simulink model "prve_riadenie"  (Simulink 7.4)
settings: Solver=ode4  StartTime=0.0  StopTime=t_sim  FixedStep=Ts  RelTol=1e-3
values from neighbouring files (symbols this model uses):
  baud = 115200    [test.m]
  com = '/dev/ttyACM0,output2.txt'    [test.m]
  D = 0    [test.m]
  fTf = 0.5    [test.m]
  fTl = 0.5    [test.m]
  fTt = 0.5    [test.m]
  I = 0    [test.m]
  P = 0    [test.m]
  Ts = 0.02    [test.m]
undefined symbols (not defined in the file or in its folder): cfan, clamp, cled, ctrltyp, insw, outsw, vstup
libraries: simulink x1, tos_lib x1
settings Model: Creator=tom  LastModifiedBy=moje
settings DataIOCC: LimitDataPoints=off  SaveOutput=off  SignalLogging=off  SaveTime=off
settings DebuggingCC: AlgebraicLoopMsg=none  ArtificialAlgebraicLoopMsg=none

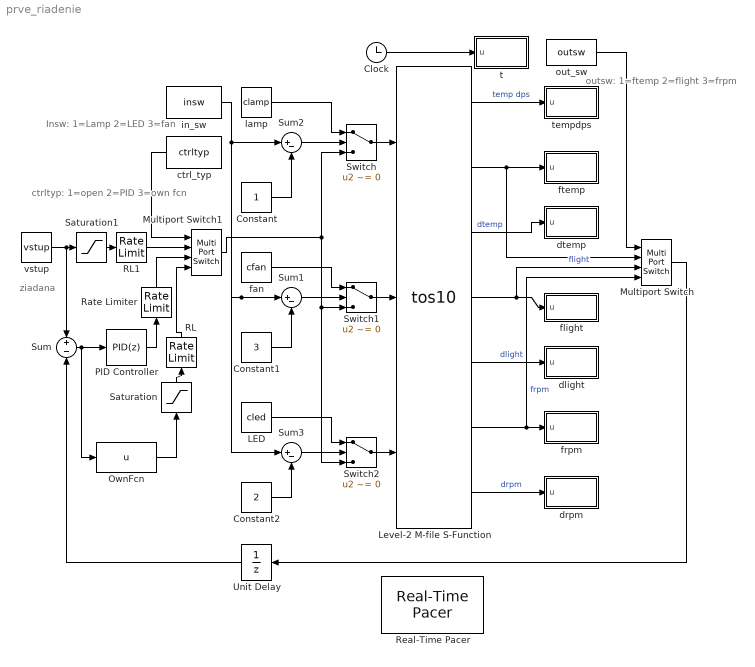
== system prve_riadenie ==
  note: ziadana
  note: Insw:
      | 1=Lamp
      | 2=LED
      | 3=fan
  note: outsw:
      | 1=ftemp
      | 2=flight
      | 3=frpm
  note: ctrltyp:
      | 1=open
      | 2=PID
      | 3=own fcn
  Clock : Clock
      settings: Decimation=10
  Constant : Constant  OutDataType=fixdt(1, 16)  OutScaling=2^0  SampleTime=Ts
  Constant1 : Constant  Value=3  OutDataType=fixdt(1, 16)  OutScaling=2^0  SampleTime=Ts
  Constant2 : Constant  Value=2  OutDataType=fixdt(1, 16)  OutScaling=2^0  SampleTime=Ts
  LED : Constant  Value=cled  SampleTime=Ts
  Level-2 M-file S-Function : M-S-Function  FunctionName=tos10  Parameters=Ts,com,baud,fTt,fTl,fTf
  Multiport Switch : MultiPortSwitch  OutDataTypeMode=double  OutDataType=fixdt(1, 16)  OutScaling=2^0  OutDataTypeStr=double  SampleTime=Ts
  Multiport Switch1 : MultiPortSwitch  OutDataTypeMode=double  OutDataType=fixdt(1, 16)  OutScaling=2^0  OutDataTypeStr=double  SampleTime=Ts
  OwnFcn : Fcn  Expr=u  SampleTime=Ts
  PID Controller : simulink/Continuous/PID Controller  DialogController=pidpack.PIDConfig.pidDDGCreate  DialogControllerArgs=DataTag0  SystemSampleTime=-1  Controller=PID  TimeDomain=Discrete-time  SampleTime=Ts  IntegratorMethod=Forward Euler  FilterMethod=Forward Euler  Form=Parallel  P=P  I=I  D=D  N=10  InitialConditionSource=internal  InitialConditionForIntegrator=0  InitialConditionForFilter=0  ExternalReset=none  LimitOutput=on  UpperSaturationLimit=100  LowerSaturationLimit=0  LinearizeAsGain=off  AntiWindupMode=clamping  Kb=10  TrackingMode=off  Kt=1  PParamMin=[]  PParamMax=[]  IParamMin=[]  IParamMax=[]  DParamMin=[]  DParamMax=[]  NParamMin=[]  NParamMax=[]  KbParamMin=[]  KbParamMax=[]  KtParamMin=[]  KtParamMax=[]  POutMin=[]  POutMax=[]  IOutMin=[]  IOutMax=[]  DOutMin=[]  DOutMax=[]  NOutMin=[]  NOutMax=[]  KbOutMin=[]  KbOutMax=[]  KtOutMin=[]  KtOutMax=[]  IntegratorOutMin=[]  IntegratorOutMax=[]  FilterOutMin=[]  FilterOutMax=[]  SumOutMin=[]  SumOutMax=[]  SumI1OutMin=[]  SumI1OutMax=[]  SumI1OutDataTypeStr=single  SumI2OutMin=[]  SumI2OutMax=[]  SumI3OutMin=[]  SumI3OutMax=[]  SumDOutMin=[]  SumDOutMax=[]  SaturationOutMin=[]  SaturationOutMax=[]  IntegratorContinuousStateAttributes=''  IntegratorStateMustResolveToSignalObject=off  IntegratorRTWStateStorageClass=Auto  FilterContinuousStateAttributes=''  FilterStateMustResolveToSignalObject=off  FilterRTWStateStorageClass=Auto
  RL : RateLimiter  RisingSlewLimit=10  FallingSlewLimit=-10  SampleTimeMode=inherited
  RL1 : RateLimiter  RisingSlewLimit=10  FallingSlewLimit=-10  SampleTimeMode=inherited
  Rate Limiter : RateLimiter  RisingSlewLimit=10  FallingSlewLimit=-10  SampleTimeMode=inherited
  Real-Time Pacer : tos_lib/Real-Time Pacer  simTimePerRealTime=1
  Saturation : Saturate  UpperLimit=100  LowerLimit=0  SampleTime=Ts  OutDataType=fixdt(1, 16)  OutScaling=2^0
  Saturation1 : Saturate  UpperLimit=100  LowerLimit=0  SampleTime=Ts  OutDataType=fixdt(1, 16)  OutScaling=2^0
  Sum : Sum  Inputs=+|-  OutDataType=fixdt(1, 16)  OutScaling=2^0  SampleTime=Ts
  Sum1 : Sum  Inputs=|+-  OutDataType=fixdt(1, 16)  OutScaling=2^0  SampleTime=Ts
  Sum2 : Sum  Inputs=|+-  OutDataType=fixdt(1, 16)  OutScaling=2^0  SampleTime=Ts
  Sum3 : Sum  Inputs=|+-  OutDataType=fixdt(1, 16)  OutScaling=2^0  SampleTime=Ts
  Switch : Switch  Criteria=u2 ~= 0  OutDataTypeMode=double  OutDataType=fixdt(1, 16)  OutScaling=2^0  OutDataTypeStr=double
  Switch1 : Switch  Criteria=u2 ~= 0  OutDataTypeMode=double  OutDataType=fixdt(1, 16)  OutScaling=2^0  OutDataTypeStr=double
  Switch2 : Switch  Criteria=u2 ~= 0  OutDataTypeMode=double  OutDataType=fixdt(1, 16)  OutScaling=2^0  OutDataTypeStr=double  SampleTime=Ts
  Unit Delay : UnitDelay  SampleTime=Ts
  ctrl_typ : Constant  Value=ctrltyp  SampleTime=Ts
  dlight : Stateflow chart  TreatAsAtomicUnit=on  SystemSampleTime=Ts
  drpm : Stateflow chart  TreatAsAtomicUnit=on  SystemSampleTime=Ts
  dtemp : Stateflow chart  TreatAsAtomicUnit=on  SystemSampleTime=Ts
  fan : Constant  Value=cfan  SampleTime=Ts
  flight : Stateflow chart  TreatAsAtomicUnit=on  SystemSampleTime=Ts
  frpm : Stateflow chart  TreatAsAtomicUnit=on  SystemSampleTime=Ts
  ftemp : Stateflow chart  TreatAsAtomicUnit=on  SystemSampleTime=Ts
  in_sw : Constant  Value=insw  SampleTime=Ts
  lamp : Constant  Value=clamp  SampleTime=Ts
  out_sw : Constant  Value=outsw  SampleTime=Ts
  t : Stateflow chart  TreatAsAtomicUnit=on  SystemSampleTime=Ts
  tempdps : Stateflow chart  TreatAsAtomicUnit=on  SystemSampleTime=Ts
  vstup : Constant  Value=vstup  SampleTime=Ts
  wires:
  lamp/1 -> Switch/1
  fan/1 -> Switch1/1
  LED/1 -> Switch2/1
  Switch/1 -> Level-2 M-file S-Function/1
  Switch1/1 -> Level-2 M-file S-Function/2
  Switch2/1 -> Level-2 M-file S-Function/3
  Sum3/1 -> Switch2/2
  Sum1/1 -> Switch1/2
  Sum2/1 -> Switch/2
  in_sw/1 -> Sum2/1, Sum1/1, Sum3/1
  Constant/1 -> Sum2/2
  Constant1/1 -> Sum1/2
  Constant2/1 -> Sum3/2
  Multiport Switch1/1 -> Switch/3, Switch1/3, Switch2/3
  vstup/1 -> Sum/1, Saturation1/1
  PID Controller/1 -> Rate Limiter/1
  Sum/1 -> PID Controller/1, OwnFcn/1
  Clock/1 -> t/1(u)
  Level-2 M-file S-Function/4 -> Multiport Switch/3, flight/1(u)  "flight"
  Level-2 M-file S-Function/5 -> dlight/1(u)  "dlight"
  Level-2 M-file S-Function/7 -> drpm/1(u)  "drpm"
  Level-2 M-file S-Function/6 -> Multiport Switch/4, frpm/1(u)  "frpm"
  Level-2 M-file S-Function/2 -> ftemp/1(u), Multiport Switch/2
  Level-2 M-file S-Function/3 -> dtemp/1(u)  "dtemp"
  Level-2 M-file S-Function/1 -> tempdps/1(u)  "temp dps"
  out_sw/1 -> Multiport Switch/1
  Multiport Switch/1 -> Unit Delay/1
  Unit Delay/1 -> Sum/2
  Rate Limiter/1 -> Multiport Switch1/3
  RL/1 -> Multiport Switch1/4
  Saturation/1 -> RL/1
  OwnFcn/1 -> Saturation/1
  ctrl_typ/1 -> Multiport Switch1/1
  Saturation1/1 -> RL1/1
  RL1/1 -> Multiport Switch1/2

== matlab function ftemp ==
  data: u input double
function fcn(u)
%#eml
eml.extrinsic('num2str');
eml.extrinsic('strcat');
eml.extrinsic('evalin');
evalin('base',strcat('ftemp(end+1)=', num2str(u),';'));
end

== matlab function tempdps ==
  data: u input double
function fcn(u)
%#eml
eml.extrinsic('num2str');
eml.extrinsic('strcat');
eml.extrinsic('evalin');
evalin('base',strcat('tempdps(end+1)=', num2str(u),';'));
end

== matlab function dtemp ==
  data: u input double
function fcn(u)
%#eml
eml.extrinsic('num2str');
eml.extrinsic('strcat');
eml.extrinsic('evalin');
evalin('base',strcat('dtemp(end+1)=', num2str(u),';'));
end

== matlab function frpm ==
  data: u input double
function fcn(u)
%#eml
eml.extrinsic('num2str');
eml.extrinsic('strcat');
eml.extrinsic('evalin');
evalin('base',strcat('frpm(end+1)=', num2str(u),';'));
end

== matlab function drpm ==
  data: u input double
function fcn(u)
%#eml
eml.extrinsic('num2str');
eml.extrinsic('strcat');
eml.extrinsic('evalin');
evalin('base',strcat('drpm(end+1)=', num2str(u),';'));
end

== matlab function flight ==
  data: u input double
function fcn(u)
%#eml
eml.extrinsic('num2str');
eml.extrinsic('strcat');
eml.extrinsic('evalin');
evalin('base',strcat('flight(end+1)=', num2str(u),';'));
end

== matlab function dlight ==
  data: u input double
function fcn(u)
%#eml
eml.extrinsic('num2str');
eml.extrinsic('strcat');
eml.extrinsic('evalin');
evalin('base',strcat('dlight(end+1)=', num2str(u),';'));
end

== matlab function t ==
  data: u input double
function fcn(u)
%#eml
eml.extrinsic('num2str');
eml.extrinsic('strcat');
eml.extrinsic('evalin');
evalin('base',strcat('t(end+1)=', num2str(u),';'));
end
